simulink model "LeastSquareMethod"  (R2021b)
settings: Solver=ode1  StartTime=0.0  StopTime=10  FixedStep=0.001  RelTol=1e-3
PostLoadFcn:
  | CCM_Parameter
libraries: simulink x1, eeGeneralControl x1
settings Model: Creator=renjianze  LastModifiedBy=renjianze
settings OptimizationCC: DefaultParameterBehavior=Inlined  EnhancedBackFolding=on  PassReuseOutputArgsAs=Individual arguments  ZeroExternalMemoryAtStartup=off  ZeroInternalMemoryAtStartup=off  OptimizeBlockOrder=speed  DifferentSizesBufferReuse=on  OptimizationCustomize=off  EfficientTunableParamExpr=on
settings DebuggingCC: ParameterTunabilityLossMsg=error
settings HardwareCC: ProdBitPerPointer=32  ProdBitPerSizeT=32  ProdBitPerPtrDiffT=32  ProdLargestAtomicInteger=Long  ProdLargestAtomicFloat=Double  ProdWordSize=32  ProdHWDeviceType=NXP->Cortex-M4
settings SFSimCC: MATLABDynamicMemAlloc=off
settings RTWCC: Description=Embedded Coder  SystemTargetFile=ert.tlc  TemplateMakefile=ert_default_tmf  CustomHeaderCode="#include  \"interface.h\""
settings CodeAppCC: ForceParamTrailComments=on  IgnoreCustomStorageClasses=off  OperatorAnnotations=on  SimulinkDataObjDesc=on  SFDataObjDesc=on  InsertBlockDesc=on
settings ERTTargetCC: TargetLangStandard=C99 (ISO)  GenerateSampleERTMain=on  InlinedParameterPlacement=NonHierarchical  ERTCustomFileTemplate=example_file_process.tlc  ERTFilePackagingFormat=Compact

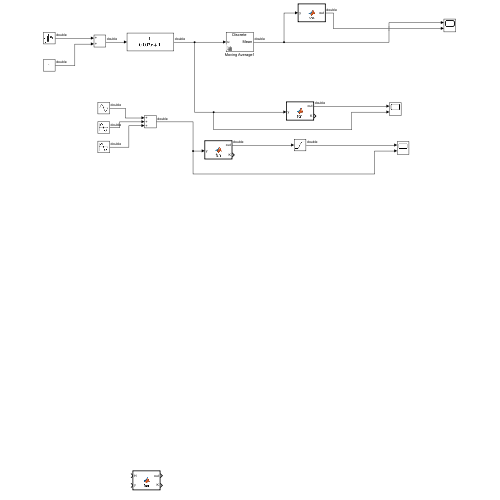
[thumbnail: Simulink's stored preview of the top-level diagram]
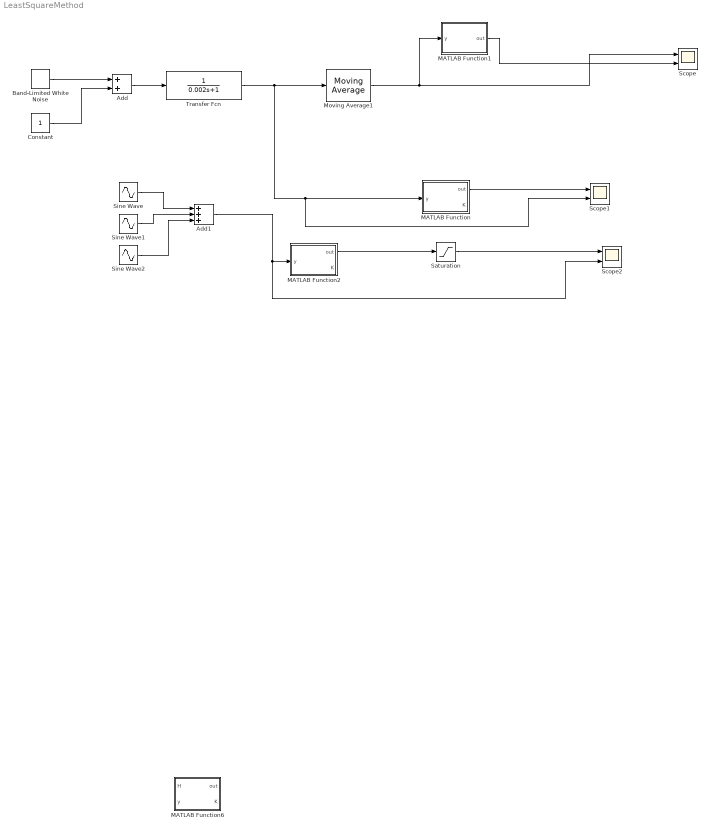
== system LeastSquareMethod ==
  Add : Sum
  Add1 : Sum  Inputs=+++
  Band-Limited White Noise : simulink/Sources/Band-Limited White Noise  Cov=[0.000002]  Ts=0.001  seed=[23341]
  Constant : Constant
  MATLAB Function : MATLAB Function  TreatAsAtomicUnit=on
  MATLAB Function1 : MATLAB Function  TreatAsAtomicUnit=on
  MATLAB Function2 : MATLAB Function  TreatAsAtomicUnit=on
  MATLAB Function6 : MATLAB Function  TreatAsAtomicUnit=on
  Moving Average1 : eeGeneralControl/Moving Average  VariantControl=Variant1  LabelModeActiveChoice=Discrete  f=50  x0=0  BufferSize=8192  Ts=0.001
      settings: SourceProductBaseCode=PS
  Saturation : Saturate  UpperLimit=20  LowerLimit=-20
  Scope : Scope  NumInputPorts=2
  Scope1 : Scope  NumInputPorts=2
  Scope2 : Scope  NumInputPorts=2
  Sine Wave : Sin  Frequency=10*2*pi  SampleTime=0
  Sine Wave1 : Sin  Amplitude=3  Frequency=20*2*pi  SampleTime=0
  Sine Wave2 : Sin  Amplitude=2  Frequency=15*2*pi  SampleTime=0
  Transfer Fcn : TransferFcn  Denominator=[0.002 1]
  wires:
  Band-Limited White Noise/1 -> Add/1
  Constant/1 -> Add/2
  Add/1 -> Transfer Fcn/1
  Transfer Fcn/1 -> Scope1/2, MATLAB Function/1(y), Moving Average1/1
  Moving Average1/1 -> MATLAB Function1/1(y), Scope/1
  MATLAB Function1/1(out) -> Scope/2
  MATLAB Function/1(out) -> Scope1/1
  Sine Wave/1 -> Add1/1
  Add1/1 -> Scope2/2, MATLAB Function2/1(y)
  MATLAB Function2/1(out) -> Saturation/1
  Saturation/1 -> Scope2/1
  Sine Wave1/1 -> Add1/2
  Sine Wave2/1 -> Add1/3

== matlab function LeastSquareMethod/MATLAB Function1 ==
  settings: updateMethod=DISCRETE
  data: y input; out output
function out = fcn(y)

persistent theta;
persistent P;
lambda = 0.5;
if isempty(theta)
    theta = 0;
end

if isempty(P)
    P = 1000;
end

P1 = P;
K = (P1*1)/(lambda + y*P1*1);

theta1 = theta;
theta = theta1+K*(y-1*theta1);

P = (1/lambda)* (P1 - K*1*P1);


out = theta;

== matlab function LeastSquareMethod/MATLAB Function ==
  settings: updateMethod=DISCRETE
  data: y input; out output; K output
function [out,K] = fcn(y)

persistent theta;
persistent P;
lambda = 0.5;
if isempty(theta)
    theta = 0;
end

if isempty(P)
    P = 1000;
end

P1 = P;
K = (P1*1)/(lambda + y*P1*1);

theta1 = theta;
theta = theta1+K*(y-1*theta1);

P = (1/lambda)* (P1 - K*1*P1);


out = theta;

== matlab function LeastSquareMethod/MATLAB Function2 ==
  settings: updateMethod=DISCRETE
  data: y input; out output; K output
function [out,K] = fcn(y)

persistent theta;
persistent P;
lambda = 0.6;
if isempty(theta)
    theta = 0;
end

if isempty(P)
    P =3000;
end

P1 = P;
K = (P1*1)/(lambda + y*P1*1);

theta1 = theta;
theta = theta1+K*(y-1*theta1);

P = (1/lambda)* (P1 - K*1*P1);


out = theta;

== matlab function LeastSquareMethod/MATLAB Function6 ==
  settings: updateMethod=DISCRETE
  data: H input; y input; out output; K output
function [out,K] = fcn(H,y)

persistent theta;
persistent P;
lambda = 0.8;
if isempty(theta)
    theta = [0;0];
end

if isempty(P)
    P = 5000*[1 0;0 1];
end



K = (P*H)*(lambda + H' * P *H)^-1;
theta = theta+K*(y-H'*theta);
P = (1/lambda)* (P - K*H'*P);


out = theta;
